simulink model "ECS_Model"  (Simulink 8.1)
settings: Solver=ode45  StartTime=0.0  StopTime=tspan(end)  RelTol=1e-3
values from neighbouring files (symbols this model uses):
  alpha = 0.2    [Config_ECS.m]    (also in Init_ECS.m)
  M8 = x(1)    [Config_ECS.m]    (also in Init_ECS.m)
  Mw1 = x(2)    [Config_ECS.m]    (also in Init_ECS.m)
  Mw2 = x(3)    [Config_ECS.m]    (also in Init_ECS.m)
  Mw3 = x(4)    [Config_ECS.m]    (also in Init_ECS.m)
  Mw4 = x(5)    [Config_ECS.m]    (also in Init_ECS.m)
  Rin1 = Rvalin/(H*L1*(1-beta1))    [Config_ECS.m]    (also in Init_ECS.m)
  Rin2 = Rvalin/(H*L2*(1-beta2))    [Config_ECS.m]    (also in Init_ECS.m)
  Rin3 = Rvalin/(H*L1*(1-beta3))    [Config_ECS.m]    (also in Init_ECS.m)
  Rin4 = Rvalin/(H*L2*(1-beta4))    [Config_ECS.m]    (also in Init_ECS.m)
  Rout1 = Rvalout/(H*L1*(1-beta1))    [Config_ECS.m]    (also in Init_ECS.m)
  Rout2 = Rvalout/(H*L2*(1-beta2))    [Config_ECS.m]    (also in Init_ECS.m)
  Rout3 = Rvalout/(H*L1*(1-beta3))    [Config_ECS.m]    (also in Init_ECS.m)
  Rout4 = Rvalout/(H*L2*(1-beta4))    [Config_ECS.m]    (also in Init_ECS.m)
  Rw1 = Rvalw/(H*L1*(1-beta1))    [Config_ECS.m]    (also in Init_ECS.m)
  Rw2 = Rvalw/(H*L2*(1-beta2))    [Config_ECS.m]    (also in Init_ECS.m)
  Rw3 = Rvalw/(H*L1*(1-beta3))    [Config_ECS.m]    (also in Init_ECS.m)
  Rw4 = Rvalw/(H*L2*(1-beta4))    [Config_ECS.m]    (also in Init_ECS.m)
  Rwin2tot = (Rvalin+Rvalgl+Rvalout)/(H*L2*beta2)    [Config_ECS.m]    (also in Init_ECS.m)
  Rwin3tot = (Rvalin+Rvalgl+Rvalout)/(H*L1*beta3)    [Config_ECS.m]    (also in Init_ECS.m)
undefined symbols (not defined in the file or in its folder): beta2, cp, cpw, H, IC, L2
libraries: simulink x6
settings Model: Creator=maasoumy  LastModifiedBy=alex  SimulationMode=accelerator
settings DataIOCC: LimitDataPoints=off  SaveFormat=StructureWithTime  SaveState=on  ReturnWorkspaceOutputs=on  OutputOption=SpecifiedOutputTimes  OutputTimes=tspan
settings DebuggingCC: StrictBusMsg=Warning

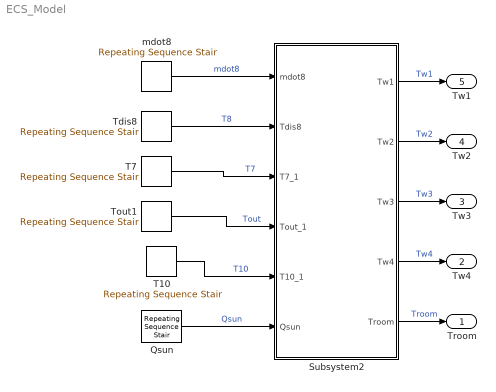
== system ECS_Model ==
  Qsun : simulink/Sources/Repeating Sequence Stair  OutValues=Qsun  tsamp=1  OutMin=[]  OutMax=[]  OutDataTypeStr=double  OutputDataTypeScalingMode=Specify via dialog  OutDataType=double  ConRadixGroup=Best Precision: Vector-wise  OutScaling=2^-12
  Subsystem2 : Subsystem
  T10 : simulink/Sources/Repeating Sequence Stair  OutValues=T10  tsamp=1  OutMin=[]  OutMax=[]  OutDataTypeStr=double  OutputDataTypeScalingMode=Specify via dialog  OutDataType=double  ConRadixGroup=Best Precision: Vector-wise  OutScaling=2^-12
  T7 : simulink/Sources/Repeating Sequence Stair  OutValues=T7  tsamp=1  OutMin=[]  OutMax=[]  OutDataTypeStr=double  OutputDataTypeScalingMode=Specify via dialog  OutDataType=double  ConRadixGroup=Best Precision: Vector-wise  OutScaling=2^-12
  Tdis8 : simulink/Sources/Repeating Sequence Stair  OutValues=Tdis8  tsamp=1  OutMin=[]  OutMax=[]  OutDataTypeStr=double  OutputDataTypeScalingMode=Specify via dialog  OutDataType=double  ConRadixGroup=Best Precision: Vector-wise  OutScaling=2^-12
  Tout1 : simulink/Sources/Repeating Sequence Stair  OutValues=Tout  tsamp=1  OutMin=[]  OutMax=[]  OutDataTypeStr=double  OutputDataTypeScalingMode=Specify via dialog  OutDataType=double  ConRadixGroup=Best Precision: Vector-wise  OutScaling=2^-12
  mdot8 : simulink/Sources/Repeating Sequence Stair  OutValues=mdot8  tsamp=1  OutMin=[]  OutMax=[]  OutDataTypeStr=double  OutputDataTypeScalingMode=Specify via dialog  OutDataType=double  ConRadixGroup=Best Precision: Vector-wise  OutScaling=2^-12
  Troom : Outport
  Tw4 : Outport  Port=2
  Tw3 : Outport  Port=3
  Tw2 : Outport  Port=4
  Tw1 : Outport  Port=5
  wires:
  Subsystem2/1(Tw1) -> Tw1/1  "Tw1"
  Subsystem2/2(Tw2) -> Tw2/1  "Tw2"
  Subsystem2/3(Tw3) -> Tw3/1  "Tw3"
  Subsystem2/4(Tw4) -> Tw4/1  "Tw4"
  Subsystem2/5(Troom) -> Troom/1  "Troom"
  mdot8/1 -> Subsystem2/1(mdot8)  "mdot8"
  Tdis8/1 -> Subsystem2/2(Tdis8)  "T8"
  T7/1 -> Subsystem2/3(T7_1)  "T7"
  Tout1/1 -> Subsystem2/4(Tout_1)  "Tout"
  T10/1 -> Subsystem2/5(T10_1)  "T10"
  Qsun/1 -> Subsystem2/6(Qsun)  "Qsun"

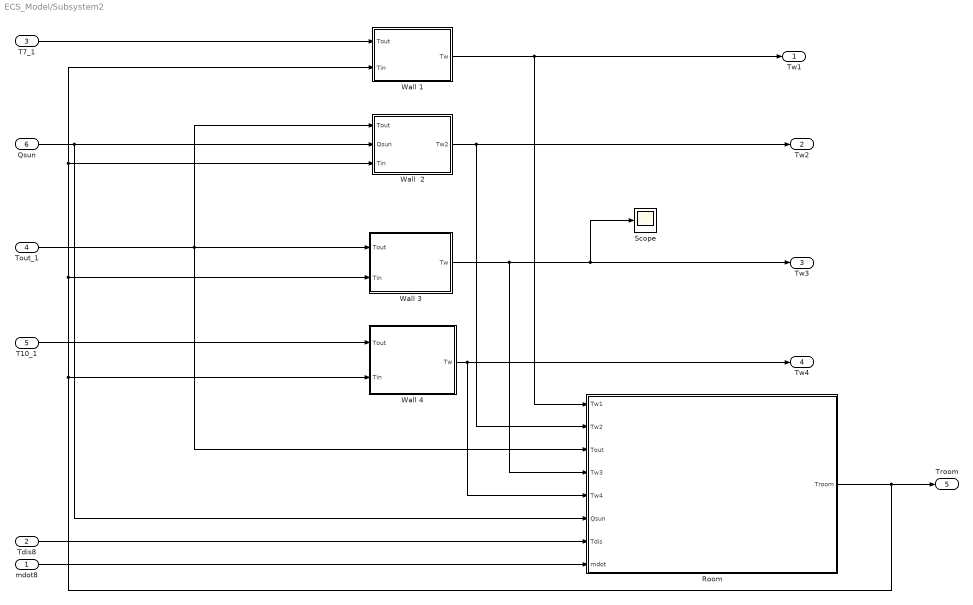
== system ECS_Model/Subsystem2 ==
  mdot8 : Inport
  Tdis8 : Inport  Port=2
  T7_1 : Inport  Port=3
  Tout_1 : Inport  Port=4
  T10_1 : Inport  Port=5
  Qsun : Inport  Port=6
  Room : Subsystem
  Scope : Scope
  Wall  2 : Subsystem
  Wall 1 : Subsystem
  Wall 3 : Subsystem
  Wall 4 : Subsystem
  Tw1 : Outport
  Tw2 : Outport  Port=2
  Tw3 : Outport  Port=3
  Tw4 : Outport  Port=4
  Troom : Outport  Port=5
  wires:
  Tout_1/1 -> Wall  2/1(Tout), Room/3(Tout), Wall 3/1(Tout)
  Wall 1/1(Tw) -> Room/1(Tw1), Tw1/1
  T7_1/1 -> Wall 1/1(Tout)
  Wall  2/1(Tw2) -> Room/2(Tw2), Tw2/1
  Wall 3/1(Tw) -> Room/4(Tw3), Scope/1, Tw3/1
  Wall 4/1(Tw) -> Room/5(Tw4), Tw4/1
  T10_1/1 -> Wall 4/1(Tout)
  Qsun/1 -> Room/6(Qsun), Wall  2/2(Qsun)
  Tdis8/1 -> Room/7(Tdis)
  mdot8/1 -> Room/8(mdot)
  Room/1(Troom) -> Wall 1/2(Tin), Wall  2/3(Tin), Wall 3/2(Tin), Wall 4/2(Tin), Troom/1

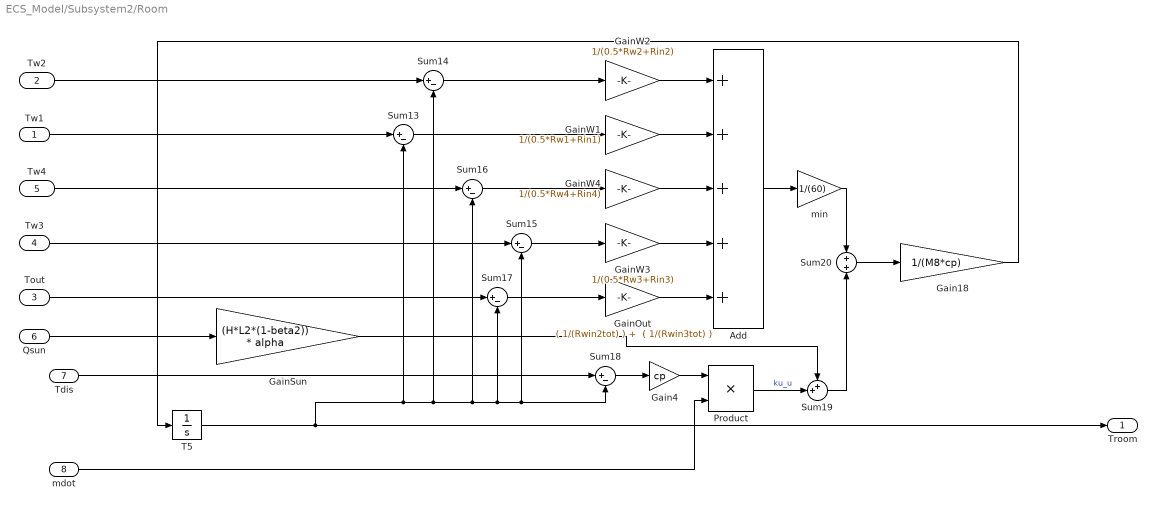
== system ECS_Model/Subsystem2/Room ==
  Tw1 : Inport
  Tw2 : Inport  Port=2
  Tout : Inport  Port=3
  Tw3 : Inport  Port=4
  Tw4 : Inport  Port=5
  Qsun : Inport  Port=6
  Tdis : Inport  Port=7
  mdot : Inport  Port=8
  Add : Sum  Inputs=+++++
  Gain18 : Gain  Gain=1/(M8*cp)
  Gain4 : Gain  Gain=cp
  GainOut : Gain  Gain="( 1/(Rwin2tot) ) +  ( 1/(Rwin3tot) )"
  GainSun : Gain  Gain=(H*L2*(1-beta2)) * alpha
  GainW1 : Gain  Gain=1/(0.5*Rw1+Rin1)
  GainW2 : Gain  Gain=1/(0.5*Rw2+Rin2)
  GainW3 : Gain  Gain=1/(0.5*Rw3+Rin3)
  GainW4 : Gain  Gain=1/(0.5*Rw4+Rin4)
  Product : Product  RndMeth=Zero
  Sum{13..18} (6 alike) : Sum  Inputs=|+-
  Sum19 : Sum  Inputs=++|
  Sum20 : Sum  Inputs=+|+
  T5 : Integrator  InitialCondition=IC(5)
  min : Gain  Gain=1/(60)
  Troom : Outport
  wires:
  Gain18/1 -> T5/1
  Sum20/1 -> Gain18/1
  min/1 -> Sum20/1
  Add/1 -> min/1
  GainW4/1 -> Add/3
  Tdis/1 -> Sum18/1
  GainW1/1 -> Add/2
  GainW2/1 -> Add/1
  Sum13/1 -> GainW1/1
  Product/1 -> Sum19/2  "ku_u"
  GainW3/1 -> Add/4
  Tw3/1 -> Sum15/1
  Tout/1 -> Sum17/1
  Tw2/1 -> Sum14/1
  Tw4/1 -> Sum16/1
  T5/1 -> Sum18/2, Sum15/2, Sum17/2, Sum16/2, Sum14/2, Sum13/2, Troom/1
  Tw1/1 -> Sum13/1
  Gain4/1 -> Product/1
  mdot/1 -> Product/2
  Sum18/1 -> Gain4/1
  Qsun/1 -> GainSun/1
  Sum15/1 -> GainW3/1
  Sum14/1 -> GainW2/1
  Sum19/1 -> Sum20/2
  Sum17/1 -> GainOut/1
  Sum16/1 -> GainW4/1
  GainOut/1 -> Add/5
  GainSun/1 -> Sum19/1

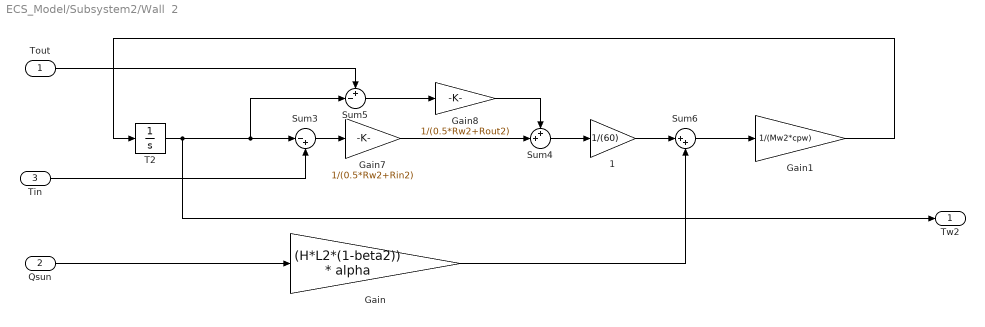
== system ECS_Model/Subsystem2/Wall  2 ==
  Tout : Inport
  Qsun : Inport  Port=2
  Tin : Inport  Port=3
  1 : Gain  Gain=1/(60)
  Gain : Gain  Gain=(H*L2*(1-beta2)) * alpha
  Gain1 : Gain  Gain=1/(Mw2*cpw)
  Gain7 : Gain  Gain=1/(0.5*Rw2+Rin2)
  Gain8 : Gain  Gain=1/(0.5*Rw2+Rout2)
  Sum3 : Sum  Inputs=|-+
  Sum4 : Sum  Inputs=++|
  Sum5 : Sum  Inputs=+-|
  Sum6 : Sum  Inputs=|++
  T2 : Integrator  InitialCondition=IC(2)
  Tw2 : Outport
  wires:
  Sum5/1 -> Gain8/1
  1/1 -> Sum6/1
  T2/1 -> Tw2/1, Sum3/1, Sum5/2
  Gain7/1 -> Sum4/2
  Sum6/1 -> Gain1/1
  Qsun/1 -> Gain/1
  Tout/1 -> Sum5/1
  Sum4/1 -> 1/1
  Sum3/1 -> Gain7/1
  Gain8/1 -> Sum4/1
  Gain1/1 -> T2/1
  Tin/1 -> Sum3/2
  Gain/1 -> Sum6/2

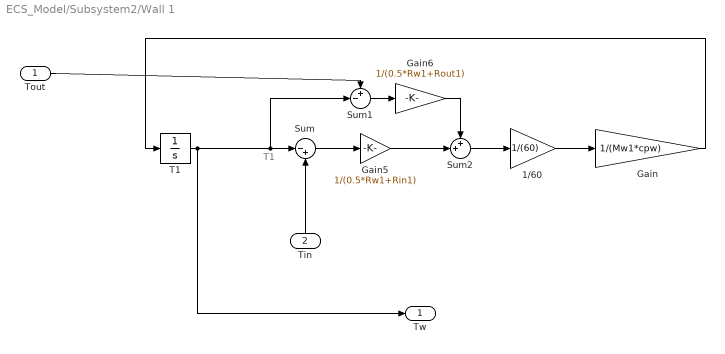
== system ECS_Model/Subsystem2/Wall 1 ==
  note: T1
  Tout : Inport
  Tin : Inport  Port=2
  1/60 : Gain  Gain=1/(60)
  Gain : Gain  Gain=1/(Mw1*cpw)
  Gain5 : Gain  Gain=1/(0.5*Rw1+Rin1)
  Gain6 : Gain  Gain=1/(0.5*Rw1+Rout1)
  Sum : Sum  Inputs=|-+
  Sum1 : Sum  Inputs=+-|
  Sum2 : Sum  Inputs=++|
  T1 : Integrator  InitialCondition=IC(1)
  Tw : Outport
  wires:
  1/60/1 -> Gain/1
  Sum2/1 -> 1/60/1
  Gain6/1 -> Sum2/1
  Gain5/1 -> Sum2/2
  Sum1/1 -> Gain6/1
  Tout/1 -> Sum1/1
  Sum/1 -> Gain5/1
  Gain/1 -> T1/1
  T1/1 -> Tw/1, Sum/1, Sum1/2
  Tin/1 -> Sum/2

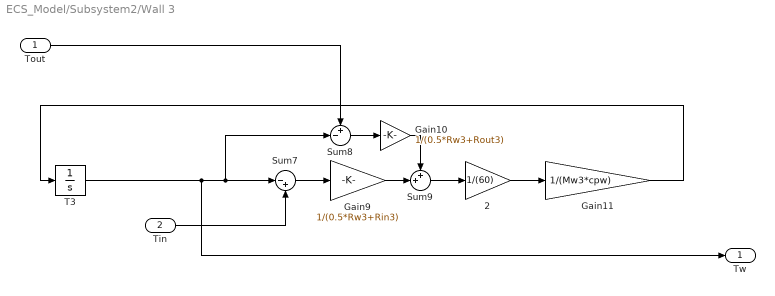
== system ECS_Model/Subsystem2/Wall 3 ==
  Tout : Inport
  Tin : Inport  Port=2
  2 : Gain  Gain=1/(60)
  Gain10 : Gain  Gain=1/(0.5*Rw3+Rout3)
  Gain11 : Gain  Gain=1/(Mw3*cpw)
  Gain9 : Gain  Gain=1/(0.5*Rw3+Rin3)
  Sum7 : Sum  Inputs=|-+
  Sum8 : Sum  Inputs=+-|
  Sum9 : Sum  Inputs=++|
  T3 : Integrator  InitialCondition=IC(3)
  Tw : Outport
  wires:
  Sum7/1 -> Gain9/1
  Sum8/1 -> Gain10/1
  Tout/1 -> Sum8/1
  T3/1 -> Tw/1, Sum8/2, Sum7/1
  Tin/1 -> Sum7/2
  Gain11/1 -> T3/1
  2/1 -> Gain11/1
  Gain9/1 -> Sum9/2
  Gain10/1 -> Sum9/1
  Sum9/1 -> 2/1

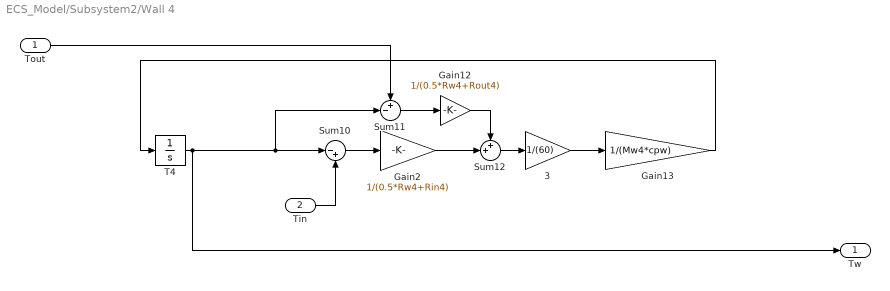
== system ECS_Model/Subsystem2/Wall 4 ==
  Tout : Inport
  Tin : Inport  Port=2
  3 : Gain  Gain=1/(60)
  Gain12 : Gain  Gain=1/(0.5*Rw4+Rout4)
  Gain13 : Gain  Gain=1/(Mw4*cpw)
  Gain2 : Gain  Gain=1/(0.5*Rw4+Rin4)
  Sum10 : Sum  Inputs=|-+
  Sum11 : Sum  Inputs=+-|
  Sum12 : Sum  Inputs=++|
  T4 : Integrator  InitialCondition=IC(4)
  Tw : Outport
  wires:
  Gain13/1 -> T4/1
  T4/1 -> Sum10/1, Sum11/2, Tw/1
  Tin/1 -> Sum10/2
  3/1 -> Gain13/1
  Sum12/1 -> 3/1
  Gain2/1 -> Sum12/2
  Gain12/1 -> Sum12/1
  Sum11/1 -> Gain12/1
  Tout/1 -> Sum11/1
  Sum10/1 -> Gain2/1
